simulink model "crazyflie_nelin_try"  (R2014b)
settings: Solver=ode45  StartTime=0.0  StopTime=100  RelTol=1e-3
values from neighbouring files (symbols this model uses):
  d = 39.73e-3    (= 0.03973)    [liniarizare_crazyflie.m]
  g = 9.81    [liniarizare_crazyflie.m]
  Ixx = 1.395e-05    [liniarizare_crazyflie.m]
  Iyy = Ixx    (= 1.395e-05)    [liniarizare_crazyflie.m]
  Izz = 2.173e-05    [liniarizare_crazyflie.m]
  m = 0.027    [liniarizare_crazyflie.m]
  Th_coef = 3.1582e-10    [liniarizare_crazyflie.m]
  Th_coefOmega_e = (omega_e-4070.3)/0.2685    (= 44702.7932961)    [liniarizare_crazyflie.m]
  To_coef = 7.9379e-12    [liniarizare_crazyflie.m]
libraries: simulink x1
settings Model: Creator=uidd7441  LastModifiedBy=uidd7441
settings DataIOCC: ExternalInput=[t,ue]  InitialState=xe

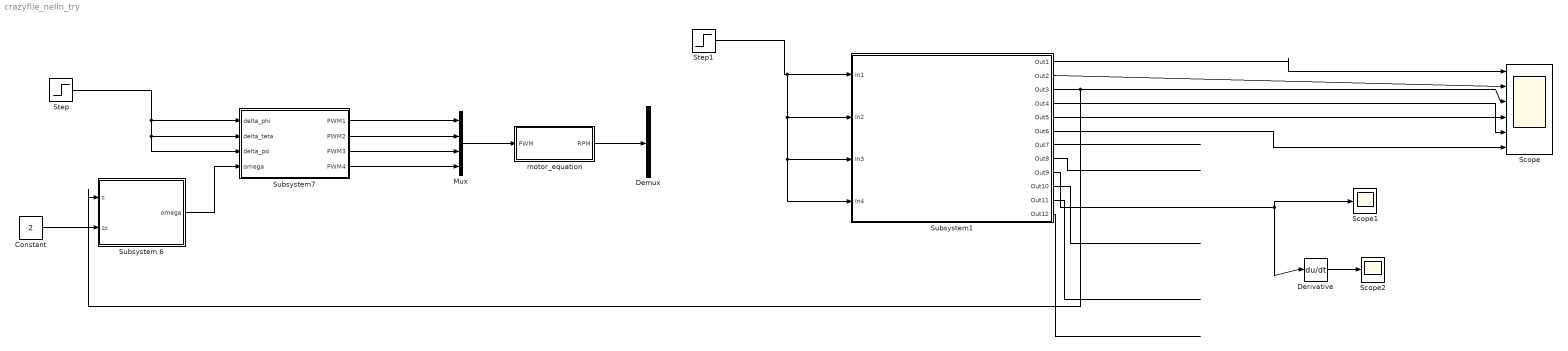
== system crazyflie_nelin_try ==
  Constant : Constant  Value=2
  Demux : Demux
  Derivative : Derivative
  Mux : Mux
  Scope : Scope  NumInputPorts=6
      settings: YMin=-300~200~-400~-4e+06~-0.5~-13  YMax=-100~600~0~0~0.5~-12
  Scope1 : Scope
      settings: SaveName=ScopeData4
  Scope2 : Scope
      settings: YMin=-1000  YMax=1000  SaveName=ScopeData5
  Step : Step  Time=0  SampleTime=0
  Step1 : Step  Time=0  After=32378  SampleTime=0
  Subsystem 6 : Subsystem
  Subsystem1 : Subsystem
  Subsystem7 : Subsystem
  motor_equation : Subsystem
  wires:
  Subsystem1/1(Out1) -> Scope/1
  Subsystem1/2(Out2) -> Scope/2
  Subsystem1/3(Out3) -> Subsystem 6/1(z), Scope/3
  Subsystem1/4(Out4) -> Scope/4
  Subsystem1/5(Out5) -> Scope/5
  Subsystem1/6(Out6) -> Scope/6
  Subsystem1/7(Out7) -> ?
  Subsystem1/8(Out8) -> ?
  Subsystem1/9(Out9) -> Derivative/1, Scope1/1
  Subsystem1/10(Out10) -> ?
  Subsystem1/11(Out11) -> ?
  Subsystem1/12(Out12) -> ?
  Derivative/1 -> Scope2/1
  motor_equation/1("RPM ") -> Demux/1
  Mux/1 -> motor_equation/1(PWM)
  Subsystem 6/1(omega) -> Subsystem7/4(omega)
  Step/1 -> Subsystem7/3(delta_psi), Subsystem7/2(delta_teta), Subsystem7/1(delta_phi)
  Subsystem7/4(PWM4) -> Mux/4
  Subsystem7/3(PWM3) -> Mux/3
  Subsystem7/2(PWM2) -> Mux/2
  Subsystem7/1(PWM1) -> Mux/1
  Constant/1 -> Subsystem 6/2(zc)
  Step1/1 -> Subsystem1/4(In4), Subsystem1/3(In3), Subsystem1/2(In2), Subsystem1/1(In1)

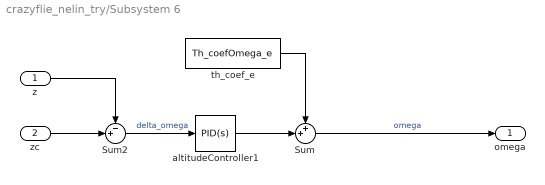
== system crazyflie_nelin_try/Subsystem 6 ==
  z : Inport
  zc : Inport  Port=2
  Sum : Sum  Inputs=++|
  Sum2 : Sum  Inputs=-+|
  altitudeController1 : simulink/Continuous/PID Controller  Controller=PID  TimeDomain=Continuous-time  SampleTime=-1  IntegratorMethod=Forward Euler  FilterMethod=Forward Euler  Form=Parallel  P=10509.4403571035  I=300.011410305238  D=33423.1282270636  N=7.7078325244016  InitialConditionSource=internal  InitialConditionForIntegrator=0  InitialConditionForFilter=0  ExternalReset=none  LimitOutput=off  UpperSaturationLimit=inf  LowerSaturationLimit=-inf  LinearizeAsGain=on  AntiWindupMode=none  Kb=1  TrackingMode=off  Kt=1  PParamMin=[]  PParamMax=[]  IParamMin=[]  IParamMax=[]  DParamMin=[]  DParamMax=[]  NParamMin=[]  NParamMax=[]  KbParamMin=[]  KbParamMax=[]  KtParamMin=[]  KtParamMax=[]  POutMin=[]  POutMax=[]  IOutMin=[]  IOutMax=[]  DOutMin=[]  DOutMax=[]  NOutMin=[]  NOutMax=[]  KbOutMin=[]  KbOutMax=[]  KtOutMin=[]  KtOutMax=[]  IntegratorOutMin=[]  IntegratorOutMax=[]  FilterOutMin=[]  FilterOutMax=[]  SumOutMin=[]  SumOutMax=[]  SumI1OutMin=[]  SumI1OutMax=[]  SumI2OutMin=[]  SumI2OutMax=[]  SumI3OutMin=[]  SumI3OutMax=[]  SumDOutMin=[]  SumDOutMax=[]  SaturationOutMin=[]  SaturationOutMax=[]  IntegratorContinuousStateAttributes=''  IntegratorStateMustResolveToSignalObject=off  IntegratorRTWStateStorageClass=Auto  FilterContinuousStateAttributes=''  FilterStateMustResolveToSignalObject=off  FilterRTWStateStorageClass=Auto  DifferentiatorICPrevScaledInput=0  DifferentiatorOutMin=[]  DifferentiatorOutMax=[]  UseFilter=on
  "th_coef_e " : Constant  Value=Th_coefOmega_e
  omega : Outport
  wires:
  "th_coef_e "/1 -> Sum/1
  Sum/1 -> omega/1  "omega"
  zc/1 -> Sum2/2
  z/1 -> Sum2/1
  Sum2/1 -> altitudeController1/1  "delta_omega"
  altitudeController1/1 -> Sum/2

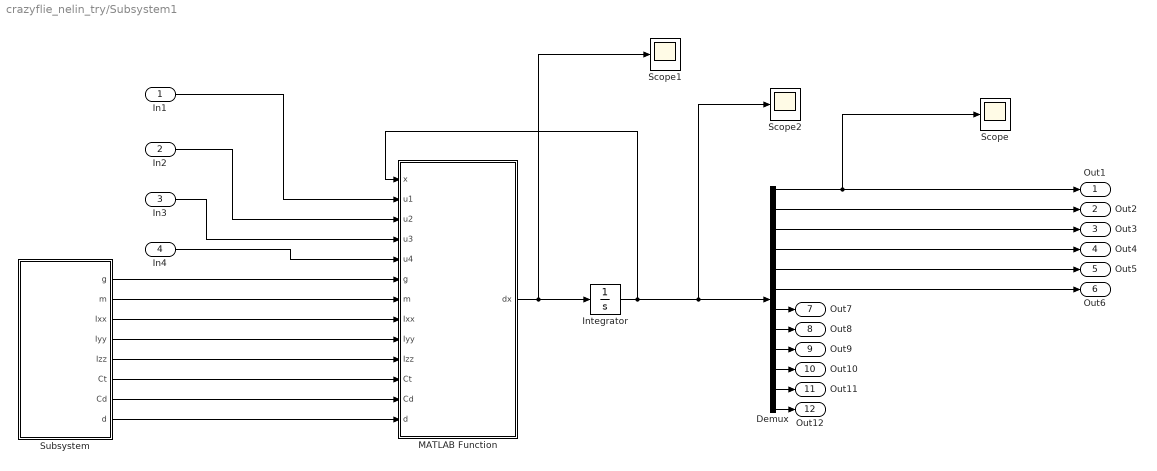
== system crazyflie_nelin_try/Subsystem1 ==
  In1 : Inport
  In2 : Inport  Port=2
  In3 : Inport  Port=3
  In4 : Inport  Port=4
  Demux : Demux  Outputs=12
  Integrator : Integrator  InitialCondition=[1 1 1 pi/3 0 0 0 0 0 0 0 0]
  MATLAB Function : MATLAB Function  TreatAsAtomicUnit=on
  Scope : Scope
  Scope1 : Scope
      settings: YMin=-4e+09  YMax=4e+09  SaveName=ScopeData2
  Scope2 : Scope
      settings: SaveName=ScopeData3
  Subsystem : Subsystem
  Out1 : Outport
  Out2 : Outport  Port=2
  Out3 : Outport  Port=3
  Out4 : Outport  Port=4
  Out5 : Outport  Port=5
  Out6 : Outport  Port=6
  Out7 : Outport  Port=7
  Out8 : Outport  Port=8
  Out9 : Outport  Port=9
  Out10 : Outport  Port=10
  Out11 : Outport  Port=11
  Out12 : Outport  Port=12
  wires:
  Demux/5 -> Out5/1
  MATLAB Function/1(dx) -> Scope1/1, Integrator/1
  Integrator/1 -> Scope2/1, Demux/1, MATLAB Function/1(x)
  Demux/2 -> Out2/1
  Demux/4 -> Out4/1
  Demux/6 -> Out6/1
  Demux/3 -> Out3/1
  Demux/1 -> Scope/1, Out1/1
  Subsystem/4(Iyy) -> MATLAB Function/9(Iyy)
  Subsystem/7(Cd) -> MATLAB Function/12(Cd)
  Subsystem/5(Izz) -> MATLAB Function/10(Izz)
  Subsystem/6(Ct) -> MATLAB Function/11(Ct)
  Subsystem/8(d) -> MATLAB Function/13(d)
  Subsystem/1(g) -> MATLAB Function/6(g)
  Subsystem/2(m) -> MATLAB Function/7(m)
  Subsystem/3(Ixx) -> MATLAB Function/8(Ixx)
  Demux/9 -> Out9/1
  Demux/11 -> Out11/1
  Demux/10 -> Out10/1
  Demux/7 -> Out7/1
  Demux/8 -> Out8/1
  Demux/12 -> Out12/1
  In1/1 -> MATLAB Function/2(u1)
  In3/1 -> MATLAB Function/4(u3)
  In2/1 -> MATLAB Function/3(u2)
  In4/1 -> MATLAB Function/5(u4)

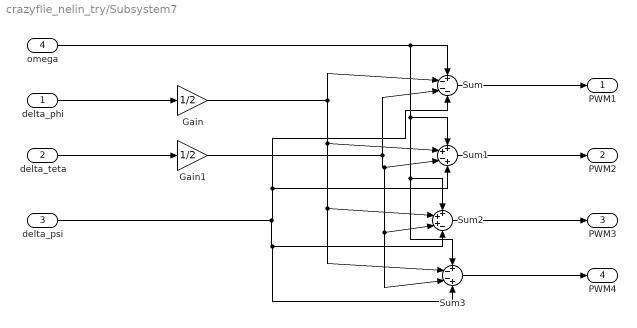
== system crazyflie_nelin_try/Subsystem7 ==
  delta_phi : Inport
  delta_teta : Inport  Port=2
  delta_psi : Inport  Port=3
  omega : Inport  Port=4
  Gain : Gain  Gain=1/2
  Gain1 : Gain  Gain=1/2
  Sum : Sum  Inputs=+---
  Sum1 : Sum  Inputs=++-+
  Sum2 : Sum  Inputs=+++-
  Sum3 : Sum  Inputs=+--+
  PWM1 : Outport
  PWM2 : Outport  Port=2
  PWM3 : Outport  Port=3
  PWM4 : Outport  Port=4
  wires:
  delta_phi/1 -> Gain/1
  delta_teta/1 -> Gain1/1
  Gain/1 -> Sum3/2, Sum2/2, Sum1/2, Sum/2
  Gain1/1 -> Sum3/3, Sum2/3, Sum1/3, Sum/3
  delta_psi/1 -> Sum3/4, Sum2/4, Sum1/4, Sum/4
  omega/1 -> Sum/1, Sum2/1, Sum3/1, Sum1/1
  Sum/1 -> PWM1/1
  Sum1/1 -> PWM2/1
  Sum2/1 -> PWM3/1
  Sum3/1 -> PWM4/1

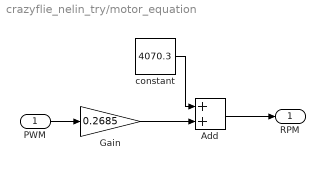
== system crazyflie_nelin_try/motor_equation ==
  PWM : Inport
  Add : Sum
  Gain : Gain  Gain=0.2685
  constant : Constant  Value=4070.3
  "RPM " : Outport
  wires:
  constant/1 -> Add/1
  Gain/1 -> Add/2
  PWM/1 -> Gain/1
  Add/1 -> "RPM "/1

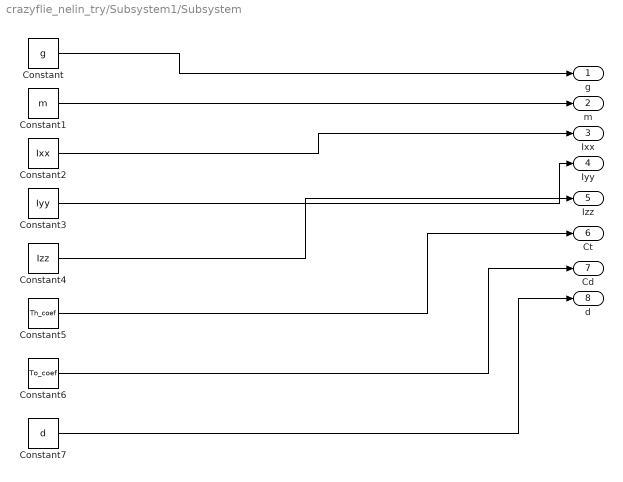
== system crazyflie_nelin_try/Subsystem1/Subsystem ==
  Constant : Constant  Value=g
  Constant1 : Constant  Value=m
  Constant2 : Constant  Value=Ixx
  Constant3 : Constant  Value=Iyy
  Constant4 : Constant  Value=Izz
  Constant5 : Constant  Value=Th_coef
  Constant6 : Constant  Value=To_coef
  Constant7 : Constant  Value=d
  g : Outport
  m : Outport  Port=2
  Ixx : Outport  Port=3
  Iyy : Outport  Port=4
  Izz : Outport  Port=5
  Ct : Outport  Port=6
  Cd : Outport  Port=7
  d : Outport  Port=8
  wires:
  Constant/1 -> g/1
  Constant5/1 -> Ct/1
  Constant4/1 -> Izz/1
  Constant7/1 -> d/1
  Constant2/1 -> Ixx/1
  Constant3/1 -> Iyy/1
  Constant1/1 -> m/1
  Constant6/1 -> Cd/1

== matlab function crazyflie_nelin_try/Subsystem1/MATLAB Function ==
  data: x input; dx output; u1 input; u2 input; u3 input; u4 input; g input; m input; Ixx input; Iyy input; Izz input; Ct input; Cd input; d input
function dx = odefun_crazyflie(x,u1,u2,u3,u4,g,m,Ixx,Iyy,Izz,Ct,Cd,d)
    
    %dx = [x y z yaw pitch roll x_rate y_rate z_rate yaw_rate pitch_rate
                %roll_rate]
    dx = zeros(size(x));
    
    Rot_InertialToBody = [cos(x(5))*cos(x(4)) cos(x(5))*sin(x(4)) -sin(x(5)); ...
    sin(x(6))*sin(x(5))*cos(x(4)) - cos(x(6))*sin(x(4)) sin(x(6))*sin(x(5))*sin(x(4)) + cos(x(6))*cos(x(4)) sin(x(6))*cos(x(5)); ...
    cos(x(6))*sin(x(5))*cos(x(4)) + sin(x(6))*sin(x(4)) cos(x(6))*sin(x(5))*sin(x(4)) - sin(x(6))*cos(x(4))  cos(x(6))*cos(x(4))];
    
    dx(1) = Rot_InertialToBody(1:3,1)'*[x(7); x(8); x(9)];
    dx(2) = Rot_InertialToBody(1:3,2)'*[x(7); x(8); x(9)];
    dx(3) = Rot_InertialToBody(1:3,3)'*[x(7); x(8); x(9)];
    
    Rot_angles = [1 sin(x(6))*tan(x(5)) cos(x(6))*tan(x(5)); ...
        0 cos(x(6)) -sin(x(6)); ...
        0 sin(x(6))/cos(x(5)) cos(x(6))/cos(x(5))];
    
    dx(6) = Rot_angles(1,1:3)*[x(12); x(11); x(10)];
    dx(5) = Rot_angles(2,1:3)*[x(12); x(11); x(10)];
    dx(4) = Rot_angles(3,1:3)*[x(12); x(11); x(10)];
    
    % Ct = thrust coeff and Cd = aerodinamical drag
    Fz = Ct*(u1^2 + u2^2 + u3^2 + u4^2);
    
    cross_prod_rate = cross([x(12); x(11); x(10)], [x(7); x(8); x(10)]);
    second_termen = Rot_InertialToBody*[0;0;g];
    
    dx(7) = - second_termen(1) - cross_prod_rate(1); 
    dx(8) = - second_termen(2) - cross_prod_rate(2); 
    dx(9) = Fz/m - second_termen(3) - cross_prod_rate(3); 
    
    Inertia_matrix = diag([Ixx Iyy Izz]);
    Mx = d*Ct/sqrt(2)*(-u1^2 - u2^2 + u3^2 + u4^2);
    My = d*Ct/sqrt(2)*(-u1^2 + u2^2 + u3^2 - u4^2);
    Mz = Cd*(-u1^2 + u2^2 - u3^2 + u4^2);
    
    Last_states = inv(Inertia_matrix)*([Mx; My; Mz] - cross([x(12); x(11); x(10)], Inertia_matrix*[x(12); x(11); x(10)]));
    dx(10) = Last_states(3);
    dx(11) = Last_states(2);
    dx(12) = Last_states(1);
    
end
